simulink model "vision_track_3_points"  (R2018b)
settings: Solver=VariableStepAuto  StartTime=0.0  StopTime=time  MaxStep=0.1  RelTol=1e-3
values from neighbouring files (symbols this model uses):
  point1 = single([x1, y1])    [Displacement_from_image.m]    (also in Measure_2_angle_from_image.m; Measure_Posotion_from_image.m; Measure_angle_from_image.m; Track_3_point.m = single(double(rgb2gray(imcrop(frame_1, [x1-template y1-templ)
  point2 = single([x2, y2])    [Measure_2_angle_from_image.m]    (also in Measure_angle_from_image.m; Track_3_point.m = single(double(rgb2gray(imcrop(frame_1, [x2-template y2-templ)
  point3 = single([x3, y3])    [Measure_2_angle_from_image.m]    (also in Measure_angle_from_image.m; Track_3_point.m = single(double(rgb2gray(imcrop(frame_1, [x3-template y3-templ)
  position1 = single(position1)    [Track_3_point.m]
  position2 = single(position2)    [Track_3_point.m]
  position3 = single(position3)    [Track_3_point.m]
undefined symbols (not defined in the file or in its folder): gray
libraries: visionanalysis x3, visiontextngfix x1, dspvision x1
settings Model: Creator=bhawnath.tiwari  LastModifiedBy=yuning.lei
settings SFSimCC: SimUseLocalCustomCode=off
settings RTWCC: RTWUseLocalCustomCode=off
settings CodeAppCC: StateflowObjectComments=on

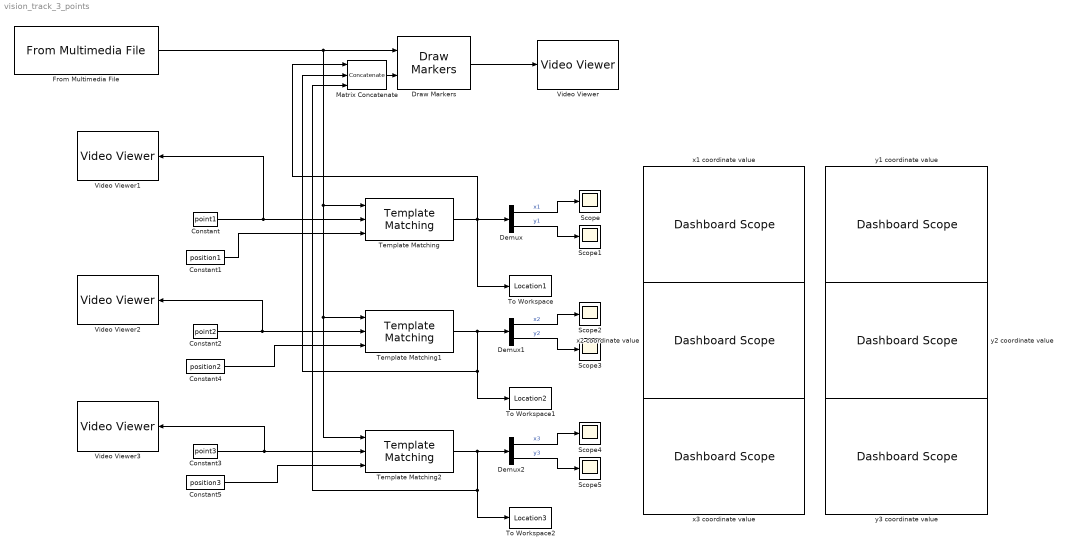
== system vision_track_3_points ==
  Constant : Constant  Value=point1
  Constant1 : Constant  Value=position1
  Constant2 : Constant  Value=point2
  Constant3 : Constant  Value=point3
  Constant4 : Constant  Value=position2
  Constant5 : Constant  Value=position3
  Demux : Demux  Outputs=2
  Demux1 : Demux  Outputs=2
  Demux2 : Demux  Outputs=2
  Draw Markers : visiontextngfix/Draw Markers  shape=Square  size=30  fill=off  fillClrSource=Specify via dialog  display=White  intensity=200  color=[200 255 100]  opacity=0.6  viewport=Entire image  antialiasing=off  inType=Obsolete  imagePorts=One multidimensional signal  prodOutputMode=Binary point scaling  prodOutputWordLength=32  prodOutputFracLength=14  memoryMode=Specify word length  memoryWordLength=16  memoryFracLength=15  roundingMode=Floor  overflowMode=off
      settings: SourceProductName=Computer Vision System Toolbox  SourceProductBaseCode=VP
  From Multimedia File : dspvision/From Multimedia File  inputFilename=g:\Utilisateurs\yuning.lei\Pictures\MEB Images\2020 07 23\mvt_perpen_10.avi  loop=on  numPlays=inf  outputStreams=Video only  videoDataType=single  audioDataType=int16  inheritSampleTime=on  userDefinedSampleTime=1/30  noAudioOutput=off  isIntensityVideo=off  fourcc=Intensity  colorVideoFormat=One multidimensional signal  outputEOF=off  dataOrg=Column-major  audioFrameSize=1024  computeAudioFrameSize=off  outSamplingMode=Sample based
      settings: SourceProductBaseCode=VP
  Matrix Concatenate : Concatenate  NumInputs=3  Mode=Multidimensional array
  Scope{,1..5} (6 alike) : Scope
  Template Matching : visionanalysis/Template Matching  metric=Sum of squared differences  output=Best match location  method=Exhaustive  nMetric=off  nSize=3  roi=on  roiValid=off  roundingMode=Floor  overflowMode=off  prodOutputMode=Binary point scaling  prodOutputWordLength=32  prodOutputFracLength=0  prodOutputSlope=2^0  accumMode=Binary point scaling  accumWordLength=32  accumFracLength=0  accumSlope=2^0  outputSlope=2^0
      settings: SourceProductName=Computer Vision System Toolbox  SourceProductBaseCode=VP
  Template Matching1 : visionanalysis/Template Matching  metric=Sum of squared differences  output=Best match location  method=Exhaustive  nMetric=off  nSize=3  roi=on  roiValid=off  roundingMode=Floor  overflowMode=off  prodOutputMode=Binary point scaling  prodOutputWordLength=32  prodOutputFracLength=0  prodOutputSlope=2^0  accumMode=Binary point scaling  accumWordLength=32  accumFracLength=0  accumSlope=2^0  outputSlope=2^0
      settings: SourceProductName=Computer Vision System Toolbox  SourceProductBaseCode=VP
  Template Matching2 : visionanalysis/Template Matching  metric=Sum of squared differences  output=Best match location  method=Exhaustive  nMetric=off  nSize=3  roi=on  roiValid=off  roundingMode=Floor  overflowMode=off  prodOutputMode=Binary point scaling  prodOutputWordLength=32  prodOutputFracLength=0  prodOutputSlope=2^0  accumMode=Binary point scaling  accumWordLength=32  accumFracLength=0  accumSlope=2^0  outputSlope=2^0
      settings: SourceProductName=Computer Vision System Toolbox  SourceProductBaseCode=VP
  To Workspace : ToWorkspace  VariableName=Location1  SampleTime=-1
      settings: Save2DSignal=2-D array (concatenate along first dimension)
  To Workspace1 : ToWorkspace  VariableName=Location2  SampleTime=-1
      settings: Save2DSignal=2-D array (concatenate along first dimension)
  To Workspace2 : ToWorkspace  VariableName=Location3  SampleTime=-1
      settings: Save2DSignal=2-D array (concatenate along first dimension)
  Video Viewer : VideoViewer  colormapValue=gray(256)  FigPos=[1922 1037 1916 929]
  Video Viewer1 : VideoViewer  FigPos=[1422 415 418 304]
  Video Viewer2 : VideoViewer  FigPos=[953 611 418 304]
  Video Viewer3 : VideoViewer  FigPos=[1431 953 418 304]
  x1 coordinate value : DashboardScope  WebBlockId=21  Ymin=770  Ymax=791
  x2 coordinate value : DashboardScope  WebBlockId=65  Ymin=770  Ymax=791
  x3 coordinate value : DashboardScope  WebBlockId=72  Ymin=770  Ymax=791
  y1 coordinate value : DashboardScope  WebBlockId=22  Ymin=330  Ymax=400
  y2 coordinate value : DashboardScope  WebBlockId=68  Ymin=330  Ymax=400
  y3 coordinate value : DashboardScope  WebBlockId=71  Ymin=330  Ymax=400
  wires:
  Constant/1 -> Video Viewer1/1, Template Matching/2
  Constant1/1 -> Template Matching/3
  Template Matching/1 -> Matrix Concatenate/1, To Workspace/1, Demux/1
  Demux/1 -> Scope/1  "x1"
  Demux/2 -> Scope1/1  "y1"
  Draw Markers/1 -> Video Viewer/1
  Template Matching1/1 -> Matrix Concatenate/2, To Workspace1/1, Demux1/1
  Demux1/2 -> Scope3/1  "y2"
  Demux1/1 -> Scope2/1  "x2"
  Demux2/2 -> Scope5/1  "y3"
  Template Matching2/1 -> Matrix Concatenate/3, To Workspace2/1, Demux2/1
  Demux2/1 -> Scope4/1  "x3"
  Constant2/1 -> Video Viewer2/1, Template Matching1/2
  Constant3/1 -> Video Viewer3/1, Template Matching2/2
  Matrix Concatenate/1 -> Draw Markers/2
  Constant4/1 -> Template Matching1/3
  Constant5/1 -> Template Matching2/3
  From Multimedia File/1 -> Template Matching2/1, Template Matching1/1, Template Matching/1, Draw Markers/1
